simulink model "InternalFaults_Winding_Delta1Delta11"  (R2015a)
settings: Solver=ode45  StartTime=0.0  StopTime=1  RelTol=1e-3
libraries: powerlib x23
settings Model: Creator=zhangtianxia  LastModifiedBy=baishuhua
settings DebuggingCC: AlgebraicLoopMsg=none  UnderspecifiedInitializationDetection=Classic  MergeDetectMultiDrivingBlocksExec=none  SolverPrmCheckMsg=warning  StateNameClashWarn=warning

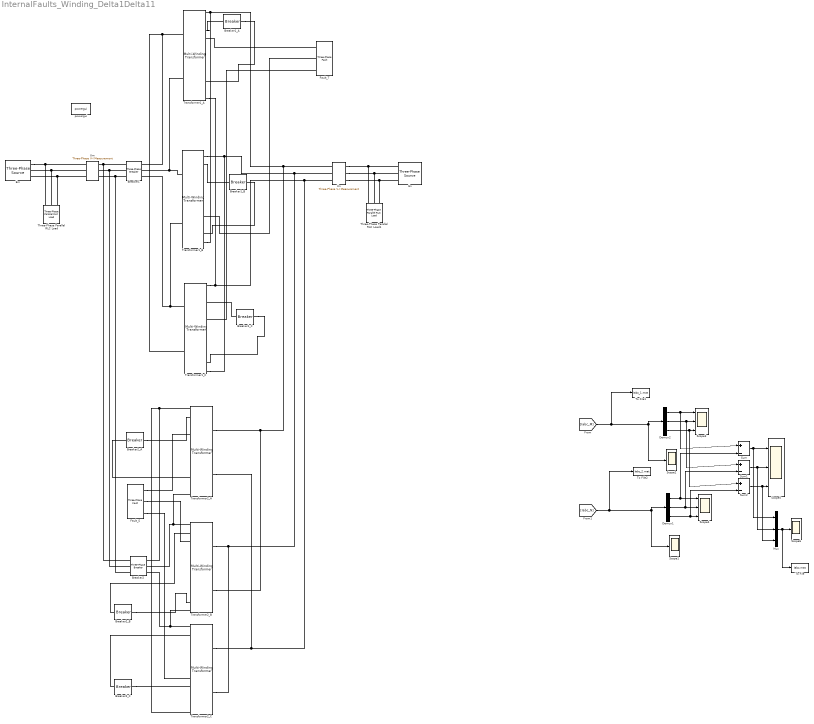
== system InternalFaults_Winding_Delta1Delta11 ==
  Breaker1 : powerlib/Elements/Three-Phase Breaker  InitialState=closed  SwitchA=on  SwitchB=on  SwitchC=on  SwitchTimes=[10 11]  External=off  BreakerResistance=0.01  SnubberResistance=1e6  SnubberCapacitance=inf  Measurements=None
  Breaker1_A : powerlib/Elements/Breaker  InitialState=0  SwitchingTimes=[0.3 0.36]  External=off  BreakerResistance=0.01  SnubberResistance=1e6  SnubberCapacitance=inf  Measurements=None  MoreParameters=on  NoBreakLoop=off
  Breaker1_B : powerlib/Elements/Breaker  InitialState=0  SwitchingTimes=[0.31 0.39]  External=off  BreakerResistance=0.01  SnubberResistance=1e6  SnubberCapacitance=inf  Measurements=None  MoreParameters=on  NoBreakLoop=off
  Breaker1_C : powerlib/Elements/Breaker  InitialState=0  SwitchingTimes=[0.41 0.49]  External=off  BreakerResistance=0.01  SnubberResistance=1e6  SnubberCapacitance=inf  Measurements=None  MoreParameters=on  NoBreakLoop=off
  Breaker2 : powerlib/Elements/Three-Phase Breaker  InitialState=open  SwitchA=off  SwitchB=off  SwitchC=off  SwitchTimes=[10 11]  External=off  BreakerResistance=0.01  SnubberResistance=1e6  SnubberCapacitance=inf  Measurements=None
  Breaker2_A : powerlib/Elements/Breaker  InitialState=0  SwitchingTimes=[10 11]  External=off  BreakerResistance=0.01  SnubberResistance=1e6  SnubberCapacitance=inf  Measurements=None  MoreParameters=on  NoBreakLoop=off
  Breaker2_B : powerlib/Elements/Breaker  InitialState=0  SwitchingTimes=[10 11]  External=off  BreakerResistance=0.01  SnubberResistance=1e6  SnubberCapacitance=inf  Measurements=None  MoreParameters=on  NoBreakLoop=off
  Breaker2_C : powerlib/Elements/Breaker  InitialState=0  SwitchingTimes=[10 11]  External=off  BreakerResistance=0.01  SnubberResistance=1e6  SnubberCapacitance=inf  Measurements=None  MoreParameters=on  NoBreakLoop=off
  Demux1 : Demux  Outputs=3
  Demux2 : Demux  Outputs=3
  Em : powerlib/Electrical Sources/Three-Phase Source  Voltage=220e3  PhaseAngle=30  Frequency=50  InternalConnection=Yg  SpecifyImpedance=off  Resistance=0.8929  Inductance=16.58e-3  ShortCircuitLevel=100e6  BaseVoltage=220e3  XRratio=7  BusType=swing  Pref=0  Qref=0  Qmin=-inf  Qmax=inf
  En : powerlib/Electrical Sources/Three-Phase Source  Voltage=500e3  PhaseAngle=10  Frequency=50  InternalConnection=Yg  SpecifyImpedance=off  Resistance=0.8929  Inductance=16.58e-3  ShortCircuitLevel=100e6  BaseVoltage=500e3  XRratio=7  BusType=swing  Pref=0  Qref=0  Qmin=-inf  Qmax=inf
  Fault_S : powerlib/Elements/Three-Phase Fault  InitialStates=0  FaultA=on  FaultB=off  FaultC=on  GroundFault=off  SwitchTimes=[10 11]  External=off  SwitchStatus=NaN  FaultResistance=0.001  GroundResistance=0.001  SnubberResistance=1e6  SnubberCapacitance=inf  Measurements=None
  Fault_T : powerlib/Elements/Three-Phase Fault  InitialStates=0  FaultA=on  FaultB=off  FaultC=on  GroundFault=off  SwitchTimes=[10 11]  External=off  SwitchStatus=NaN  FaultResistance=0.001  GroundResistance=0.001  SnubberResistance=1e6  SnubberCapacitance=inf  Measurements=None
  Mux : Mux  Inputs=3
  Scope1 : Scope
      settings: TickLabels=on  TimeRange=0.1599999999999999  YMin=-50  YMax=450  MaxDataPoints=50000
  Scope2 : Scope
      settings: TickLabels=on  TimeRange=0.1599999999999999  YMin=-50  YMax=450  MaxDataPoints=50000
  Scope3 : Scope  NumInputPorts=3
      settings: TickLabels=on  TimeRange=0.1599999999999999  YMin=-50~-500~-50  YMax=450~50~450  SaveName=ScopeData2  MaxDataPoints=50000
  Scope4 : Scope  NumInputPorts=3
      settings: TickLabels=on  TimeRange=0.1599999999999999  YMin=-50~-500~-50  YMax=450~50~450  SaveName=ScopeData3  MaxDataPoints=50000
  Scope5 : Scope  NumInputPorts=3
      settings: TickLabels=on  TimeRange=0.1599999999999999  YMin=-50~-500~-50  YMax=450~50~450  SaveName=ScopeData4  MaxDataPoints=50000
  Scope6 : Scope
      settings: TickLabels=on  TimeRange=0.1599999999999999  YMin=-50  YMax=450  SaveName=ScopeData5  MaxDataPoints=50000
  Sum : Sum  Inputs=|+-
  Sum1 : Sum  Inputs=|+-
  Sum2 : Sum  Inputs=|+-
  Three-Phase Parallel RLC Load : powerlib/Elements/Three-Phase Parallel RLC Load  LConnTagsString=A|B|C  Configuration=Y (grounded)  NominalVoltage=220e3  NominalFrequency=50  ActivePower=10e6  InductivePower=100  CapacitivePower=100  Measurements=None  LoadType=constant Z
  Three-Phase Parallel RLC Load1 : powerlib/Elements/Three-Phase Parallel RLC Load  LConnTagsString=A|B|C  Configuration=Y (grounded)  NominalVoltage=500e3  NominalFrequency=50  ActivePower=10e6  InductivePower=100  CapacitivePower=100  Measurements=None  LoadType=constant Z
  To File : ToFile  Filename=Iabc.mat  MatrixName=Iabc  SaveFormat=Timeseries
  To File1 : ToFile  Filename=Iabc_1.mat  MatrixName=Iabc_1  SaveFormat=Timeseries
  To File2 : ToFile  Filename=Iabc_2.mat  MatrixName=Iabc_2  SaveFormat=Timeseries
  Transformer1_A : powerlib/Elements/Multi-Winding Transformer  LeftWindings=1  RightWindings=1  TappedWindings=taps on upper right winding  NumberOfTaps=9  UNITS=pu  NominalPower=[100e6 50]  NominalVoltages=[ 220e3 500e3 ]  WindingResistances="[ 0.005  0.005]"  WindingInductances="[ 0.02  0.02]"  SetSaturation=on  Rm=50  Lm=50  Saturation=[ 0,0 ; 0.0024,1.2 ; 1.0,1.52 ]  Hysteresis=off  DataFile='hysteresis.mat'  Measurements=None  MoreParameters=off  BreakLoop=off  DataType=off  InitialFlux=-791.797657006776  TransfoNumber=1
  Transformer1_B : powerlib/Elements/Multi-Winding Transformer  LeftWindings=1  RightWindings=1  TappedWindings=taps on upper right winding  NumberOfTaps=9  UNITS=pu  NominalPower=[100e6 50]  NominalVoltages=[ 220e3 500e3 ]  WindingResistances="[ 0.005  0.005]"  WindingInductances="[ 0.02  0.02]"  SetSaturation=on  Rm=50  Lm=50  Saturation=[ 0,0 ; 0.0024,1.2 ; 1.0,1.52 ]  Hysteresis=off  DataFile='hysteresis.mat'  Measurements=None  MoreParameters=off  BreakLoop=off  DataType=off  InitialFlux=339.875727811436  TransfoNumber=1
  Transformer1_C : powerlib/Elements/Multi-Winding Transformer  LeftWindings=1  RightWindings=1  TappedWindings=taps on upper right winding  NumberOfTaps=9  UNITS=pu  NominalPower=[100e6 50]  NominalVoltages=[220e3 500e3]  WindingResistances="[ 0.005  0.005]"  WindingInductances="[ 0.02  0.02]"  SetSaturation=on  Rm=50  Lm=50  Saturation=[ 0,0 ; 0.0024,1.2 ; 1.0,1.52 ]  Hysteresis=off  DataFile='hysteresis.mat'  Measurements=None  MoreParameters=off  BreakLoop=off  DataType=off  InitialFlux=451.921929193185  TransfoNumber=1
  Transformer2_A : powerlib/Elements/Multi-Winding Transformer  LeftWindings=1  RightWindings=1  TappedWindings=taps on upper left winding  NumberOfTaps=9  UNITS=pu  NominalPower=[100e6 50]  NominalVoltages=[ 220e3 500e3 ]  WindingResistances="[ 0.005  0.005]"  WindingInductances="[ 0.02  0.02]"  SetSaturation=on  Rm=50  Lm=50  Saturation=[ 0,0 ; 0.0024,1.2 ; 1.0,1.52 ]  Hysteresis=off  DataFile='hysteresis.mat'  Measurements=None  MoreParameters=off  BreakLoop=off  DataType=off  InitialFlux=-89.2467125575992  TransfoNumber=1
  Transformer2_B : powerlib/Elements/Multi-Winding Transformer  LeftWindings=1  RightWindings=1  TappedWindings=taps on upper left winding  NumberOfTaps=9  UNITS=pu  NominalPower=[100e6 50]  NominalVoltages=[ 220e3 500e3 ]  WindingResistances="[ 0.005  0.005]"  WindingInductances="[ 0.02  0.02]"  SetSaturation=on  Rm=50  Lm=50  Saturation=[ 0,0 ; 0.0024,1.2 ; 1.0,1.52 ]  Hysteresis=off  DataFile='hysteresis.mat'  Measurements=None  MoreParameters=off  BreakLoop=off  DataType=off  InitialFlux=65.9235667652752  TransfoNumber=1
  Transformer2_C : powerlib/Elements/Multi-Winding Transformer  LeftWindings=1  RightWindings=1  TappedWindings=taps on upper left winding  NumberOfTaps=9  UNITS=pu  NominalPower=[100e6 50]  NominalVoltages=[ 220e3 500e3 ]  WindingResistances="[ 0.005  0.005]"  WindingInductances="[ 0.02  0.02]"  SetSaturation=on  Rm=50  Lm=50  Saturation=[ 0,0 ; 0.0024,1.2 ; 1.0,1.52 ]  Hysteresis=off  DataFile='hysteresis.mat'  Measurements=None  MoreParameters=off  BreakLoop=off  DataType=off  InitialFlux=23.3231457911869  TransfoNumber=1
  Um : powerlib/Measurements/Three-Phase V-I Measurement  VoltageMeasurement=no  SetLabelV=off  LabelV=Vabc  Vpu=off  VpuLL=off  CurrentMeasurement=yes  SetLabelI=on  LabelI=Iabc_M  Ipu=on  Pbase=100e6  Vbase=220e3  OutputType=Complex  PhasorSimulation=off  PSBequivalent=0
  Un : powerlib/Measurements/Three-Phase V-I Measurement  VoltageMeasurement=no  SetLabelV=off  LabelV=Vabc  Vpu=off  VpuLL=off  CurrentMeasurement=yes  SetLabelI=on  LabelI=Iabc_N  Ipu=on  Pbase=100e6  Vbase=500e3  OutputType=Complex  PhasorSimulation=off  PSBequivalent=0
  powergui : powerlib/powergui  Priority=1  SimulationMode=Discrete  SolverType=Tustin  SampleTime=1e-4  frequency=60  SPID=off  DisableSnubberDevices=off  DisableRonSwitches=off  DisableVfSwitches=off  SwTol=0  DisplayEquations=off  Interpol=off  methode=off  Ts=0  FunctionMessages=off  echomessages=off  HookPort=off  EnableUseOfTLC=off  x0status=blocks  frequencyindice=50  Pbase=100e6  ErrMax=1e-4  Iterations=50  UnitsV=kV  UnitsW=MW  buscounter=0  RestoreLinks=warning  ResistiveCurrentMeasurement=off  Frange=[0:2:500]  Ylog=off  Xlog=on  ShowGrid=off  save=off  variable=ZData  structure=ScopeData  ZoomFFT=off  StartTime=0.191  cycles=2  DisplayStyle=5  fundamental=50  FreqAxis=on  MaxFrequency=250  frequencyindicesteady=1  RmsSteady=1  display=off
  wires:
  Demux2/1 -> Sum/1, Scope3/1
  Demux2/2 -> Sum1/1, Scope3/2
  Demux2/3 -> Sum2/1, Scope3/3
  [Iabc_M] -> To File1/1, Demux2/1, Scope2/1
  Demux1/1 -> Sum/2, Scope4/1
  Demux1/2 -> Sum1/2, Scope4/2
  Demux1/3 -> Sum2/2, Scope4/3
  Sum/1 -> Mux/1, Scope5/1
  Sum1/1 -> Mux/2, Scope5/2
  Sum2/1 -> Mux/3, Scope5/3
  Mux/1 -> To File/1, Scope6/1
  [Iabc_N] -> To File2/1, Demux1/1, Scope1/1
  connections:
  Em/RConn1 -- Um/LConn1 -- Three-Phase Parallel RLC Load/LConn1
  Three-Phase Parallel RLC Load/LConn2 -- Um/LConn2 -- Em/RConn2
  Three-Phase Parallel RLC Load/LConn3 -- Um/LConn3 -- Em/RConn3
  Un/RConn1 -- En/RConn1 -- Three-Phase Parallel RLC Load1/LConn1
  Un/RConn2 -- En/RConn2 -- Three-Phase Parallel RLC Load1/LConn2
  Un/RConn3 -- En/RConn3 -- Three-Phase Parallel RLC Load1/LConn3
  Transformer1_A/LConn1 -- Transformer1_C/LConn2 -- Breaker1/RConn1
  Transformer1_B/LConn1 -- Transformer1_A/LConn2 -- Breaker1/RConn2
  Transformer1_C/LConn1 -- Transformer1_B/LConn2 -- Breaker1/RConn3
  Transformer1_A/RConn1 -- Transformer1_B/RConn11 -- Transformer2_B/RConn2 -- Transformer2_A/RConn1 -- Un/LConn1
  Transformer1_B/RConn1 -- Transformer1_C/RConn11 -- Transformer2_C/RConn2 -- Transformer2_B/RConn1 -- Un/LConn2
  Transformer1_C/RConn1 -- Transformer1_A/RConn11 -- Transformer2_A/RConn2 -- Transformer2_C/RConn1 -- Un/LConn3
  Breaker1/LConn1 -- Breaker2/LConn1 -- Um/RConn1
  Breaker1/LConn2 -- Breaker2/LConn2 -- Um/RConn2
  Breaker1/LConn3 -- Breaker2/LConn3 -- Um/RConn3
  Transformer2_A/LConn1 -- Transformer2_C/LConn11 -- Breaker2/RConn1
  Transformer2_B/LConn1 -- Transformer2_A/LConn11 -- Breaker2/RConn2
  Transformer2_C/LConn1 -- Transformer2_B/LConn11 -- Breaker2/RConn3
  Breaker1_B/RConn1 -- Transformer1_B/RConn10
  Breaker2_A/LConn1 -- Transformer2_A/LConn2
  Breaker2_B/LConn1 -- Transformer2_B/LConn10
  Breaker2_B/RConn1 -- Transformer2_B/LConn2
  Breaker2_C/LConn1 -- Transformer2_C/LConn8
  Transformer2_A/LConn9 -- Breaker2_A/RConn1
  Breaker1_C/RConn1 -- Transformer1_C/RConn10
  Breaker1_C/LConn1 -- Transformer1_C/RConn3
  Transformer1_A/RConn3 -- Breaker1_A/LConn1
  Breaker1_A/RConn1 -- Transformer1_A/RConn9
  Fault_T/LConn1 -- Transformer1_A/RConn4
  Fault_S/LConn1 -- Transformer2_A/LConn4
  Transformer1_B/RConn2 -- Breaker1_B/LConn1
  Fault_S/LConn2 -- Transformer2_B/LConn3
  Fault_T/LConn2 -- Transformer1_B/RConn8
  Breaker2_C/RConn1 -- Transformer2_C/LConn2
  Fault_S/LConn3 -- Transformer2_C/LConn7
  Fault_T/LConn3 -- Transformer1_C/RConn5
